simulink model "ocena_7"  (R2019b)
settings: Solver=FixedStepDiscrete  StartTime=0.0  StopTime=inf  FixedStep=SampleTime  RelTol=1e-3  EnableMultiTasking=on
PreLoadFcn:
  | SampleTime = 1/500;
  | 
  | q0 = [0 0 0 0 0 0];
  | 
  | system('MotomanVodenje.exe &')
undefined symbols (not defined in the file): DiscIntNeverNeededParam
libraries: simulink x2, dspinverses x1, xpcutilitieslib x1, dspnetwork x1
settings Model: EnablePacing=on  Creator=Martina Loknar  LastModifiedBy=student
settings DataIOCC: LimitDataPoints=on  SaveFormat=Array  ReturnWorkspaceOutputs=off
settings OptimizationCC: LifeSpan=inf
settings DebuggingCC: SolverPrmCheckMsg=warning  ParameterPrecisionLossMsg=none  SFUnexpectedBacktrackingDiag=warning  SFNoUnconditionalDefaultTransitionDiag=warning  SFExecutionAtInitializationDiag=none  ArithmeticOperatorsInVariantConditions=warning
settings HardwareCC: ProdBitPerPointer=32  ProdBitPerSizeT=32  ProdBitPerPtrDiffT=32  ProdLargestAtomicFloat=None  ProdIntDivRoundTo=Undefined  ProdEndianess=Unspecified  ProdWordSize=32  ProdHWDeviceType=32-bit Generic
settings ModelReferenceCC: PropagateSignalLabelsOutOfModel=off
settings SFSimCC: SimUseLocalCustomCode=off  CustomCodeUndefinedFunction=UseInterfaceOnly
settings RTWCC: RTWUseLocalCustomCode=off
settings CodeAppCC: StateflowObjectComments=on
settings GRTTargetCC: TargetLangStandard=C89/C90 (ANSI)  GeneratePreprocessorConditionals=Disable all
settings ConfigComp: CovMetricSettings=dw  CovHtmlReporting=on  CovSaveCumulativeToWorkspaceVar=on  CovSaveSingleToWorkspaceVar=on  CovExternalEMLEnable=off  CovSFcnEnable=off

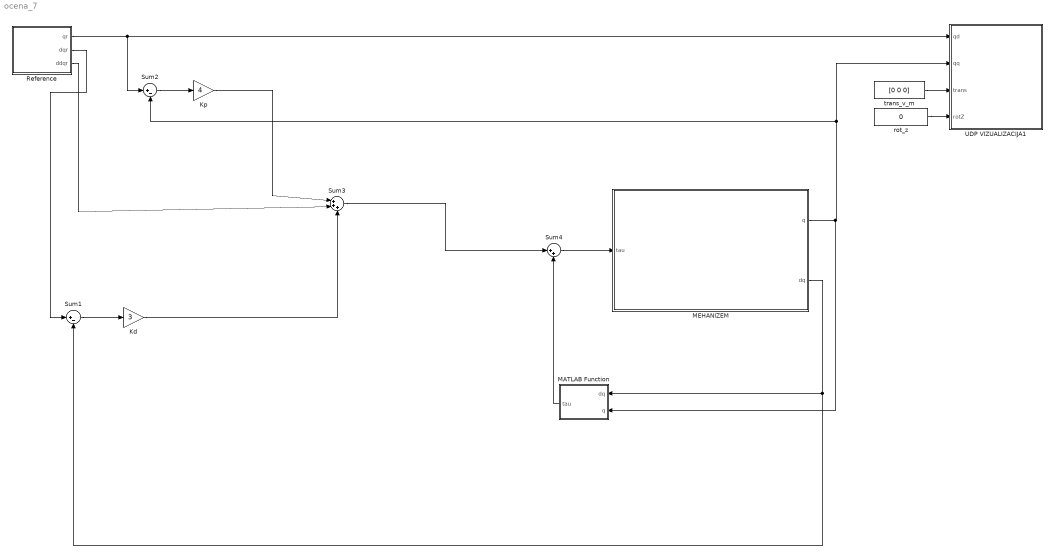
== system ocena_7 ==
  Kd : Gain  Gain=3
  "Kp " : Gain  Gain=4
  MATLAB Function : MATLAB Function  TreatAsAtomicUnit=on
  MEHANIZEM : Subsystem
  Reference : Subsystem  mask{reference=Min Jerk Trajectory}
      mask TypeOptions reference: Constant | Min Jerk Trajectory
  Sum1 : Sum  Inputs=|+-
  Sum2 : Sum  Inputs=|+-
  Sum3 : Sum  Inputs=|+++
  Sum4 : Sum  Inputs=|++
  UDP VIZUALIZACIJA1 : Subsystem
  rot_z : Constant  Value=0
  trans_v_m : Constant  Value=[0 0 0]
  wires:
  trans_v_m/1 -> UDP VIZUALIZACIJA1/3(trans)
  rot_z/1 -> UDP VIZUALIZACIJA1/4(rotZ)
  Reference/1(qr) -> Sum2/1, UDP VIZUALIZACIJA1/1(qd)
  MEHANIZEM/1(q) -> MATLAB Function/2(q), Sum2/2, UDP VIZUALIZACIJA1/2(qq)
  Reference/2(dqr) -> Sum1/1
  MEHANIZEM/2(dq) -> MATLAB Function/1(dq), Sum1/2
  Sum1/1 -> Kd/1
  Sum2/1 -> "Kp "/1
  "Kp "/1 -> Sum3/1
  Kd/1 -> Sum3/3
  Reference/3(ddqr) -> Sum3/2
  Sum4/1 -> MEHANIZEM/1(tau)
  MATLAB Function/1(tau) -> Sum4/2
  Sum3/1 -> Sum4/1

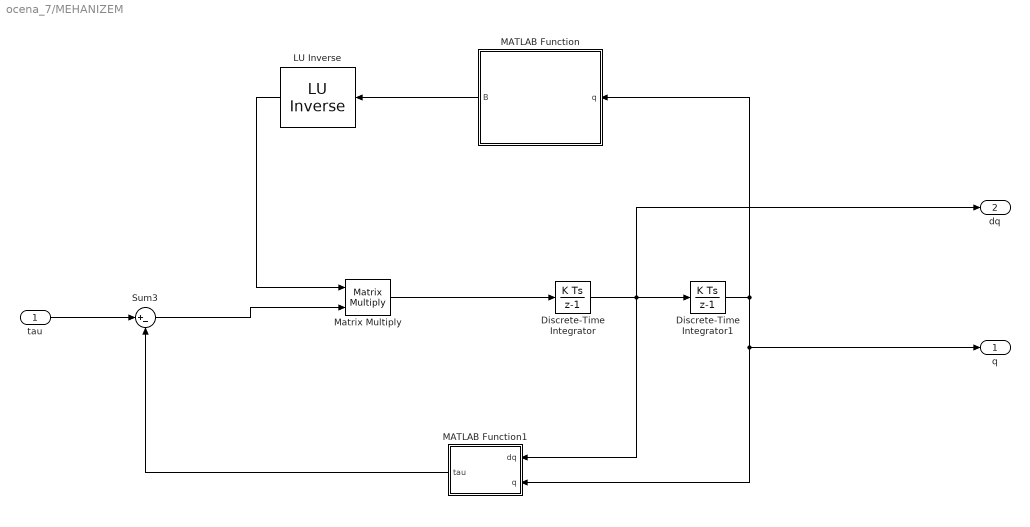
== system ocena_7/MEHANIZEM ==
  tau : Inport
  " LU Inverse" : dspinverses/ LU Inverse
      settings: SourceProductName=DSP System Toolbox
  Discrete-Time Integrator : DiscreteIntegrator  InitialCondition=[0;0;0;0;0;0]  SampleTime=1/500  ICPrevOutput=DiscIntNeverNeededParam  ICPrevScaledInput=DiscIntNeverNeededParam
  Discrete-Time Integrator1 : DiscreteIntegrator  InitialCondition=[0;0;0;0;0;0]  SampleTime=1/500  ICPrevOutput=DiscIntNeverNeededParam  ICPrevScaledInput=DiscIntNeverNeededParam
  MATLAB Function : MATLAB Function  TreatAsAtomicUnit=on
  MATLAB Function1 : MATLAB Function  TreatAsAtomicUnit=on
  Matrix Multiply : Product  Multiplication=Matrix(*)
  Sum3 : Sum  Inputs=|+-
  q : Outport
  dq : Outport  Port=2
  wires:
  Sum3/1 -> Matrix Multiply/2
  " LU Inverse"/1 -> Matrix Multiply/1
  Discrete-Time Integrator/1 -> dq/1, MATLAB Function1/1(dq), Discrete-Time Integrator1/1
  MATLAB Function1/1(tau) -> Sum3/2
  MATLAB Function/1(B) -> " LU Inverse"/1
  Matrix Multiply/1 -> Discrete-Time Integrator/1
  Discrete-Time Integrator1/1 -> q/1, MATLAB Function1/2(q), MATLAB Function/1(q)
  tau/1 -> Sum3/1

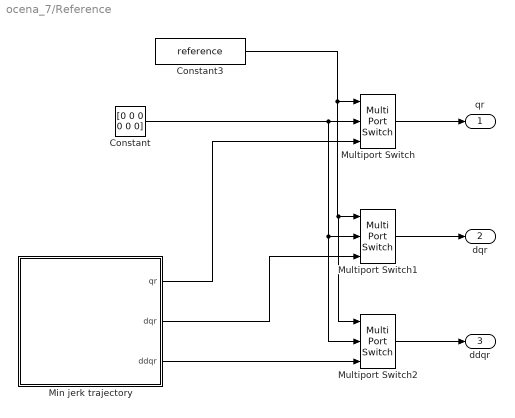
== system ocena_7/Reference ==
  Constant : Constant  Value=[0 0 0 0 0 0]
  Constant3 : Constant  Value=reference
  Min jerk trajectory : Subsystem
  Multiport Switch : MultiPortSwitch  Inputs=2
  Multiport Switch1 : MultiPortSwitch  Inputs=2
  Multiport Switch2 : MultiPortSwitch  Inputs=2
  qr : Outport
  dqr : Outport  Port=2
  ddqr : Outport  Port=3
  wires:
  Constant3/1 -> Multiport Switch2/1, Multiport Switch1/1, Multiport Switch/1
  Constant/1 -> Multiport Switch1/2, Multiport Switch2/2, Multiport Switch/2
  Multiport Switch/1 -> qr/1
  Multiport Switch1/1 -> dqr/1
  Multiport Switch2/1 -> ddqr/1
  Min jerk trajectory/1(qr) -> Multiport Switch/3
  Min jerk trajectory/2(dqr) -> Multiport Switch1/3
  Min jerk trajectory/3(ddqr) -> Multiport Switch2/3

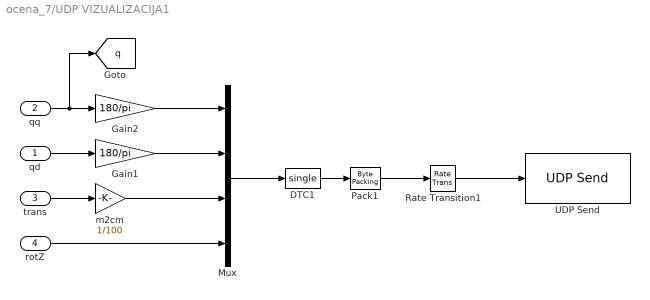
== system ocena_7/UDP VIZUALIZACIJA1 ==
  qd : Inport
  qq : Inport  Port=2
  trans : Inport  Port=3
  rotZ : Inport  Port=4
  DTC1 : DataTypeConversion  OutDataTypeStr=single
  Gain1 : Gain  Gain=180/pi
  Gain2 : Gain  Gain=180/pi
  Mux : Mux
  Pack1 : xpcutilitieslib/Byte Packing   MaskPackedDataType=uint8  MaskUnpackedDataTypes={'single'}  MaskAlignment=1
  Rate Transition1 : RateTransition
  UDP Send : dspnetwork/UDP Send  remoteURL='127.0.0.1'  remotePort=25300  localURL='0.0.0.0'  localPortSource=Automatically determine  localPort=-1  sampletime=-1  blockPlatform=[]  separateLengthPort=0
      settings: SourceProductName=Simulink
  m2cm : Gain  Gain=1/100
  tag scope: q=global
  wires:
  DTC1/1 -> Pack1/1
  Pack1/1 -> Rate Transition1/1
  Rate Transition1/1 -> UDP Send/1
  trans/1 -> m2cm/1
  Mux/1 -> DTC1/1
  m2cm/1 -> Mux/3
  rotZ/1 -> Mux/4
  qq/1 -> [q], Gain2/1
  qd/1 -> Gain1/1
  Gain2/1 -> Mux/1
  Gain1/1 -> Mux/2

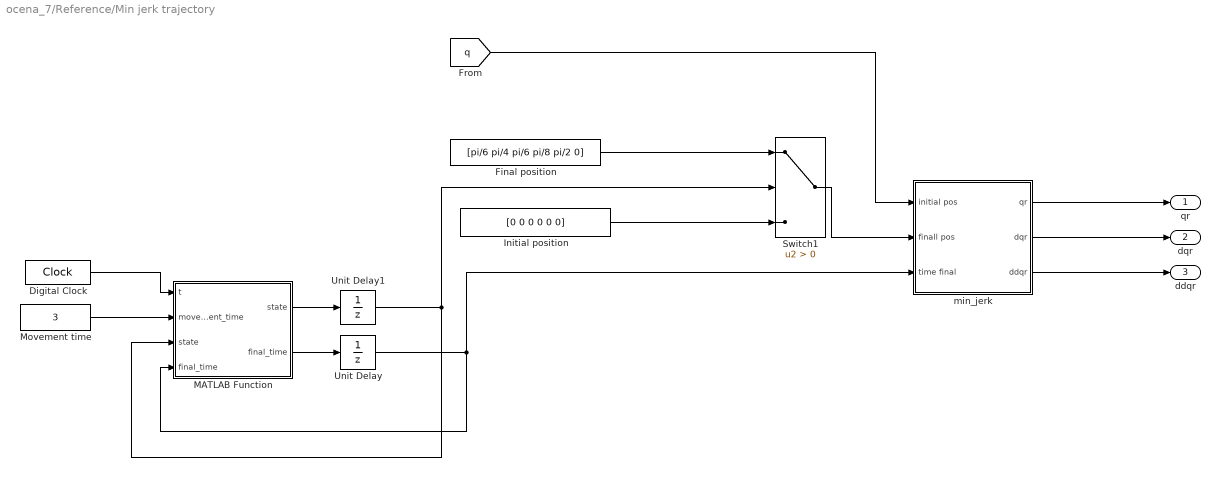
== system ocena_7/Reference/Min jerk trajectory ==
  Digital Clock : DigitalClock  SampleTime=SampleTime
  Final position : Constant  Value=[pi/6 pi/4 pi/6 pi/8 pi/2 0]
  Initial position : Constant  Value=[0 0 0 0 0 0]
  MATLAB Function : MATLAB Function  TreatAsAtomicUnit=on
  Movement time : Constant  Value=3
  Switch1 : Switch  Criteria=u2 > Threshold
  Unit Delay : UnitDelay  InitialCondition=10  SampleTime=-1  HasFrameUpgradeWarning=on
  Unit Delay1 : UnitDelay  InitialCondition=1  SampleTime=-1  HasFrameUpgradeWarning=on
  min_jerk : Subsystem
  qr : Outport
  dqr : Outport  Port=2
  ddqr : Outport  Port=3
  wires:
  [q] -> min_jerk/1(initial pos)
  Digital Clock/1 -> MATLAB Function/1(t)
  MATLAB Function/2(final_time) -> Unit Delay/1
  min_jerk/3(ddqr) -> ddqr/1
  Movement time/1 -> MATLAB Function/2(movement_time)
  min_jerk/1(qr) -> qr/1
  min_jerk/2(dqr) -> dqr/1
  MATLAB Function/1(state) -> Unit Delay1/1
  Unit Delay1/1 -> MATLAB Function/3("state "), Switch1/2
  Initial position/1 -> Switch1/3
  Unit Delay/1 -> MATLAB Function/4("final_time "), min_jerk/3(time final)
  Final position/1 -> Switch1/1
  Switch1/1 -> min_jerk/2(finall pos)

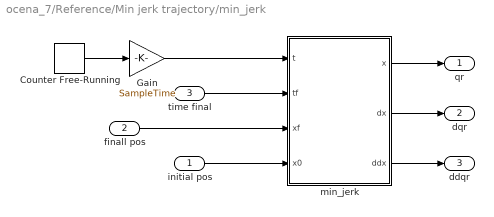
== system ocena_7/Reference/Min jerk trajectory/min_jerk ==
  initial pos : Inport
  finall pos : Inport  Port=2
  time final : Inport  Port=3
  Counter Free-Running : simulink/Sources/Counter Free-Running  NumBits=32  tsamp=-1
  Gain : Gain  Gain=SampleTime
  min_jerk : Subsystem
  qr : Outport
  dqr : Outport  Port=2
  ddqr : Outport  Port=3
  wires:
  Gain/1 -> min_jerk/1(t)
  time final/1 -> min_jerk/2(tf)
  finall pos/1 -> min_jerk/3(xf)
  Counter Free-Running/1 -> Gain/1
  min_jerk/1(x) -> qr/1
  initial pos/1 -> min_jerk/4(x0)
  min_jerk/2(dx) -> dqr/1
  min_jerk/3(ddx) -> ddqr/1

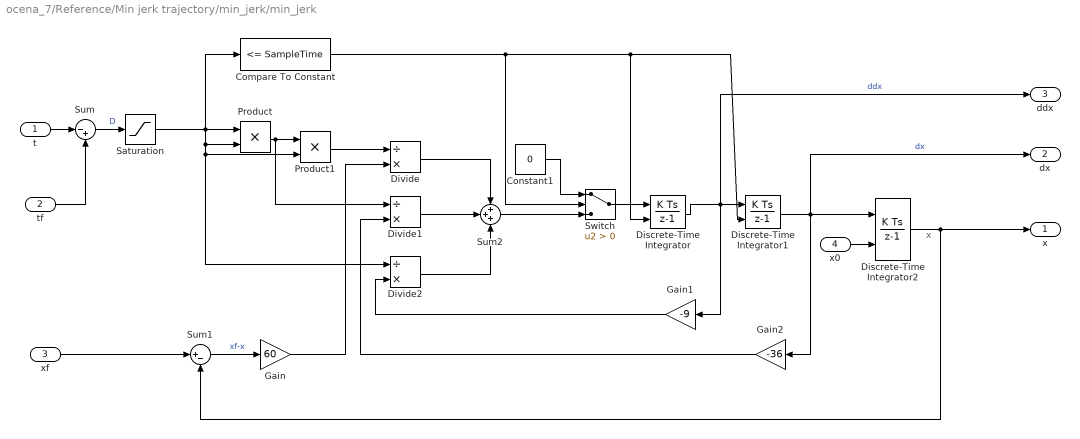
== system ocena_7/Reference/Min jerk trajectory/min_jerk/min_jerk ==
  note: x
  t : Inport
  tf : Inport  Port=2
  xf : Inport  Port=3
  x0 : Inport  Port=4
  Compare To Constant : simulink/Logic and Bit Operations/Compare To Constant  relop=<=  const=SampleTime  OutDataTypeStr=uint8  ZeroCross=off
  Constant1 : Constant  Value=0
  Discrete-Time Integrator : DiscreteIntegrator  ExternalReset=rising  SampleTime=SampleTime  ICPrevOutput=DiscIntNeverNeededParam  ICPrevScaledInput=DiscIntNeverNeededParam
  Discrete-Time Integrator1 : DiscreteIntegrator  ExternalReset=rising  SampleTime=SampleTime  ICPrevOutput=DiscIntNeverNeededParam  ICPrevScaledInput=DiscIntNeverNeededParam
  Discrete-Time Integrator2 : DiscreteIntegrator  InitialConditionSource=external  InitialCondition=[-0.1 -0.1 -0.1]  SampleTime=SampleTime  ICPrevOutput=DiscIntNeverNeededParam  ICPrevScaledInput=DiscIntNeverNeededParam
  Divide : Product  Inputs=/*
  Divide1 : Product  Inputs=/*
  Divide2 : Product  Inputs=/*
  Gain : Gain  Gain=60
  Gain1 : Gain  Gain=-9
  Gain2 : Gain  Gain=-36
  Product : Product  RndMeth=Zero
  Product1 : Product  RndMeth=Zero
  Saturation : Saturate  UpperLimit=inf  LowerLimit=SampleTime
  Sum : Sum  Inputs=|-+
  Sum1 : Sum  Inputs=|+-
  Sum2 : Sum  Inputs=+++
  Switch : Switch  Criteria=u2 > Threshold
  x : Outport
  dx : Outport  Port=2
  ddx : Outport  Port=3
  wires:
  Sum/1 -> Saturation/1  "D"
  Discrete-Time Integrator/1 -> ddx/1, Discrete-Time Integrator1/1, Gain1/1  "ddx"
  Discrete-Time Integrator1/1 -> dx/1, Discrete-Time Integrator2/1, Gain2/1  "dx"
  Discrete-Time Integrator2/1 -> x/1, Sum1/2
  xf/1 -> Sum1/1
  Sum1/1 -> Gain/1  "xf-x"
  Product/1 -> Product1/1, Divide1/1
  Product1/1 -> Divide/1
  Gain/1 -> Divide/2
  Gain2/1 -> Divide1/2
  Gain1/1 -> Divide2/2
  Divide1/1 -> Sum2/2
  Divide2/1 -> Sum2/3
  Divide/1 -> Sum2/1
  Saturation/1 -> Product/1, Product/2, Product1/2, Divide2/1, Compare To Constant/1
  Compare To Constant/1 -> Discrete-Time Integrator/2, Discrete-Time Integrator1/2, Switch/2
  Sum2/1 -> Switch/3
  Switch/1 -> Discrete-Time Integrator/1
  Constant1/1 -> Switch/1
  t/1 -> Sum/1
  tf/1 -> Sum/2
  x0/1 -> Discrete-Time Integrator2/2

== matlab function ocena_7/MATLAB Function ==
  data: tau output; dq input; q input
function tau = torque(dq, q)

ddp0 = [0,0,9.81]';
ddq = zeros(6,1);  

tau = torque(ddq, dq, q, ddp0);

== matlab function ocena_7/MEHANIZEM/MATLAB Function ==
  data: q input; B output
function B = inertia6(q)

    B = inertia6(q);
end

== matlab function ocena_7/MEHANIZEM/MATLAB Function1 ==
  data: dq input; tau output; q input
function tau = tau6_q_dq(dq, q)

tau = tau6_q_dq(dq, q);

== matlab function ocena_7/Reference/Min jerk trajectory/MATLAB Function ==
  data: t input; state output; movement_time input; state input; final_time input; final_time output
function [state, final_time] = ch_dir(t, movement_time, state, final_time)

if (mod(t, movement_time)==0)
    if (state==1)
        state = 0;
    else
        state = 1;
    end
    final_time = t + movement_time;
end
